simulink library "Ground_Storage"  (Simulink 8.2)
settings: Solver=ode45  StartTime=0.0  StopTime=10.0  RelTol=1e-3
libraries: carnot x2
settings Model: Creator=lena.frank  LastModifiedBy=drhf

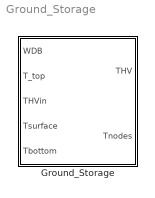
== system Ground_Storage ==
  Ground_Storage : Subsystem  mask(ground storage){xs=10, ys=10, zs=5, ground=clay (humid), fill=clay (humid), dp=0.1, kp=0.001, zp=1, np=20, t0=20, refine=1, mpts=5}
      mask prompts: xs "extension perpendicular to pipes [m]"; ys "extension parallel to pipes [m]"; zs "depth of storage [m]"; fill "filling"; dp "diameter of pipe [m]"; kp "roughness of pipe [m]"; zp "depth of pipe [m]"; np "number of pipes"; t0 "initial temperature [degree centigrade]"; refine "refine factor"; mpts "number of measurement points"
      mask help:
      | Three-dimensional ground storage model.
      | Look under mask to change the surface model.
      mask init:
      | xs = max(xs, 0.001);
      | ys = max(ys, 0.001);
      | zp = max(zp, 0.001);
      | zs = max(zs, zp);
      | np = max(0, np);
      | dp = max(dp, 0.001);
      | kp = max(kp, 0.001);
      | cond=[0.7 1.88 1.45 2.9 1.28];
      | lg = cond(ground);
      | cap = [1382400 1798200 2410560  2864160 1933800];
      | cg = cap(ground);
      | lf = cond(fill);
      | cf = cap(fill);
      mask Help: web(fullfile(path_carnot('help'),'Ground_Storage.html'),'-helpbrowser')
      mask TypeOptions ground: sand (dry) | sand (saturated with water) | clay (humid) | clay (saturated with water)
      mask TypeOptions fill: sand (dry) | sand (saturated with water) | clay (humid) | clay (saturated with water) | concrete
      mask TypeOptions refine: 1 | 2 | 3 | 4 | 6 | 8 | 10 | 16 | 24 | 32
      mask Display: plot(0,0,100,100,[30,60,70,40,30],[70,70,80,80,70],[68,59,56,59,56,52,48,51,48,44,40,44,41,32],[83,72,72,78,78,72,72,78,78,72,72,78,78,67],[61,58,44,31,30],[69,60,56,60,67],[62,60,52,37,29,29],[68,56,47,48,57,67],[64,67,67,65,57,44,32,27,28],[71,62,53,43,35,35,40,54,66])

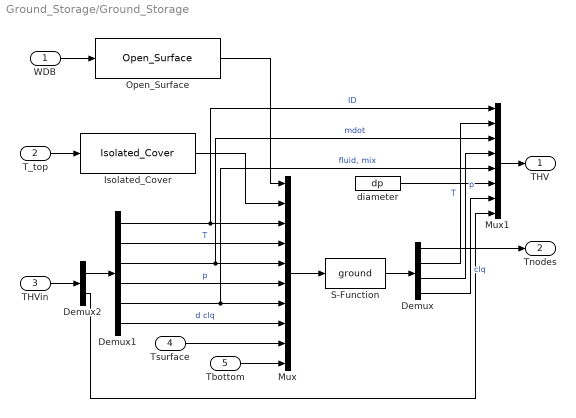
== system Ground_Storage/Ground_Storage ==
  WDB : Inport
  T_top : Inport  Port=2
  THVin : Inport  Port=3
  Tsurface : Inport  Port=4
  Tbottom : Inport  Port=5
  Demux : Demux  Outputs=[3*mpts 1 1 3]
  Demux1 : Demux  Outputs=[1 1 1 1 2 4]
  Demux2 : Demux  Outputs=[10 10]
  Isolated_Cover : carnot/Storage/Thermal/surface_models/Isolated_Cover  u=0.6
  Mux : Mux  Inputs=10
  Mux1 : Mux  Inputs=8
  Open_Surface : carnot/Storage/Thermal/surface_models/Open_Surface  albedo=0.6
  S-Function : S-Function  FunctionName=ground  Parameters=xs, ys, zs, cg, lg, dp, kp, np, zp, cf, lf, t0, refine, mpts  EnableBusSupport=off
  diameter : Constant  Value=dp
  THV : Outport
  Tnodes : Outport  Port=2
  wires:
  Demux/4 -> Mux1/7  "clq"
  Demux2/2 -> Mux1/8
  Demux2/1 -> Demux1/1
  THVin/1 -> Demux2/1
  Demux1/2 -> Mux/4  "T"
  Demux1/4 -> Mux/6  "p"
  Demux1/6 -> Mux/8  "d clq"
  Demux1/3 -> Mux/5, Mux1/3  "mdot"
  Demux1/5 -> Mux/7, Mux1/5  "fluid, mix"
  Tsurface/1 -> Mux/9
  Tbottom/1 -> Mux/10
  Demux/1 -> Tnodes/1
  Mux1/1 -> THV/1
  Demux/2 -> Mux1/2  "T"
  Demux/3 -> Mux1/4  "p"
  Mux/1 -> S-Function/1
  diameter/1 -> Mux1/6
  WDB/1 -> Open_Surface/1
  Open_Surface/1 -> Mux/1
  Isolated_Cover/1 -> Mux/2
  Demux1/1 -> Mux1/1, Mux/3  "ID"
  S-Function/1 -> Demux/1
  T_top/1 -> Isolated_Cover/1
